simulink model "Lecture_4_Exercises_Simulink"  (R2023b)
settings: Solver=ode1  StartTime=0.0  StopTime=10  FixedStep=0.01  RelTol=1e-3
values from neighbouring files (symbols this model uses):
  A = [-0.4, 0, -0.01 ... (first row only)    [Lecture_4_Exercises.m]
  B = [6.3 ... (first row only)    [Lecture_4_Exercises.m]
  C = eye(size(A))    [Lecture_4_Exercises.m]
  D = zeros(size(B))    [Lecture_4_Exercises.m]
  K = place(A, B, lambda_cl)    [Lecture_4_Exercises.m]
undefined symbols (not defined in the file or in its folder): init_cond, K_lqr, K_lqr_d, T, u_star, x_star
settings Model: Creator=therk  LastModifiedBy=therk

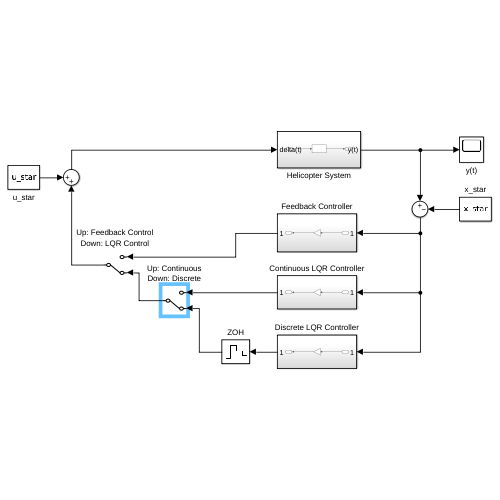
[thumbnail: Simulink's stored preview of the top-level diagram]
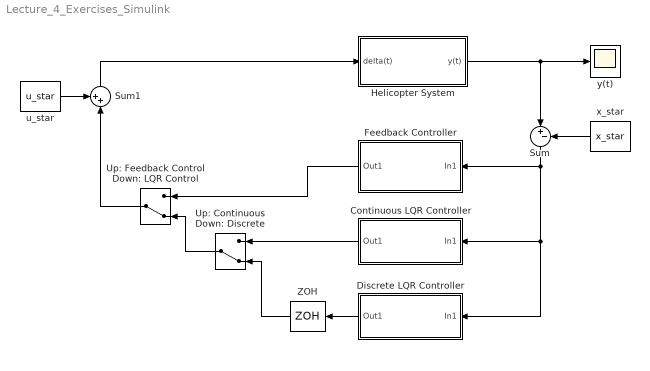
== system Lecture_4_Exercises_Simulink ==
  Continuous LQR Controller : Subsystem
  Discrete LQR Controller : Subsystem
  Feedback Controller : Subsystem
  Helicopter System : Subsystem
  Sum : Sum  Inputs=|+-
  Sum1 : Sum  Inputs=++|
  Up: Continuous Down: Discrete : ManualSwitch  CurrentSetting=0
  Up: Feedback Control Down: LQR Control : ManualSwitch  CurrentSetting=0
  ZOH : ZeroOrderHold  SampleTime=T
  u_star : Constant  Value=u_star
  x_star : Constant  Value=x_star
  y(t) : Scope
  wires:
  Helicopter System/1(y(t)) -> y(t)/1, Sum/1
  Sum/1 -> Discrete LQR Controller/1(In1), Continuous LQR Controller/1(In1), Feedback Controller/1(In1)
  Up: Feedback Control Down: LQR Control/1 -> Sum1/2
  x_star/1 -> Sum/2
  Sum1/1 -> Helicopter System/1(delta(t))
  u_star/1 -> Sum1/1
  Feedback Controller/1(Out1) -> Up: Feedback Control Down: LQR Control/1
  Continuous LQR Controller/1(Out1) -> Up: Continuous Down: Discrete/1
  Discrete LQR Controller/1(Out1) -> ZOH/1
  Up: Continuous Down: Discrete/1 -> Up: Feedback Control Down: LQR Control/2
  ZOH/1 -> Up: Continuous Down: Discrete/2

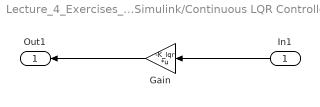
== system Lecture_4_Exercises_Simulink/Continuous LQR Controller ==
  In1 : Inport
  Gain : Gain  Gain=-K_lqr  Multiplication=Matrix(K*u)
  Out1 : Outport
  wires:
  In1/1 -> Gain/1
  Gain/1 -> Out1/1

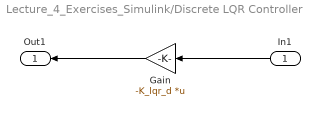
== system Lecture_4_Exercises_Simulink/Discrete LQR Controller ==
  In1 : Inport
  Gain : Gain  Gain=-K_lqr_d  Multiplication=Matrix(K*u)
  Out1 : Outport
  wires:
  In1/1 -> Gain/1
  Gain/1 -> Out1/1

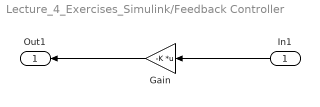
== system Lecture_4_Exercises_Simulink/Feedback Controller ==
  In1 : Inport
  Gain : Gain  Gain=-K  Multiplication=Matrix(K*u)
  Out1 : Outport
  wires:
  In1/1 -> Gain/1
  Gain/1 -> Out1/1

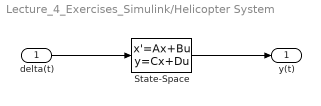
== system Lecture_4_Exercises_Simulink/Helicopter System ==
  delta(t) : Inport
  State-Space : StateSpace  A=A  B=B  C=C  D=D  InitialCondition=init_cond
  y(t) : Outport
  wires:
  delta(t)/1 -> State-Space/1
  State-Space/1 -> y(t)/1
